simulink model "dsogi_3phpll"  (R2024b)
settings: configuration reference "CONFI" (kept outside this file)
InitFcn:
  | gain_vac=1/(220*sqrt(2));
values from neighbouring files (symbols this model uses):
  cos_th = cos(2*pi*50*t)    [fidelity_pfc_vals.m]
  sin_th = sin(2*pi*50*t)    [fidelity_pfc_vals.m]
  ts = 0.0001    [dic_pfc3ph.sldd]    (also in dictionary.sldd)
  tsw = 1/(fsw*1e3)    (= 1.53846153846e-05)    [fidelity_pfc_vals.m]
undefined symbols (not defined in the file or in its folder): DiscIntNeverNeededParam
libraries: simulink x5, dspswit3 x1, mcbcontrolslib x1
settings Model: DataDictionary=dic_pfc3ph.sldd  Creator=Angel  LastModifiedBy=Angel
settings ConfigSetRef: SourceName=CONFI

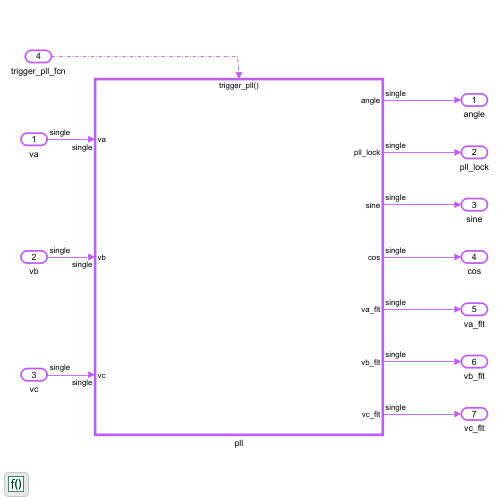
[thumbnail: Simulink's stored preview of the top-level diagram]
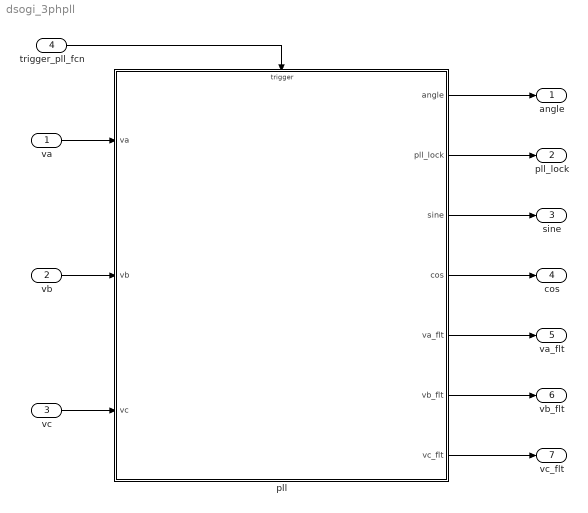
== system dsogi_3phpll ==
  va : Inport  OutDataTypeStr=single
  vb : Inport  Port=2  OutDataTypeStr=single
  vc : Inport  Port=3  OutDataTypeStr=single
  trigger_pll_fcn : Inport  Port=4  OutDataTypeStr=single  OutputFunctionCall=on
  pll : Subsystem
      settings: RTWSystemCode=Inline  RTWFcnNameOpts=Use subsystem name  RTWFileNameOpts=Use subsystem name  RTWMemSecFuncInitTerm=Default  RTWMemSecFuncExecute=Default
  angle : Outport
  pll_lock : Outport  Port=2
  sine : Outport  Port=3
  cos : Outport  Port=4
  va_flt : Outport  Port=5
  vb_flt : Outport  Port=6
  vc_flt : Outport  Port=7
  wires:
  trigger_pll_fcn/1 -> pll/Trigger
  pll/5(va_flt) -> va_flt/1
  va/1 -> pll/1(va)
  pll/2(pll_lock) -> pll_lock/1
  pll/3(sine) -> sine/1
  pll/4(cos) -> cos/1
  vb/1 -> pll/2(vb)
  vc/1 -> pll/3(vc)
  pll/1(angle) -> angle/1
  pll/7(vc_flt) -> vc_flt/1
  pll/6(vb_flt) -> vb_flt/1

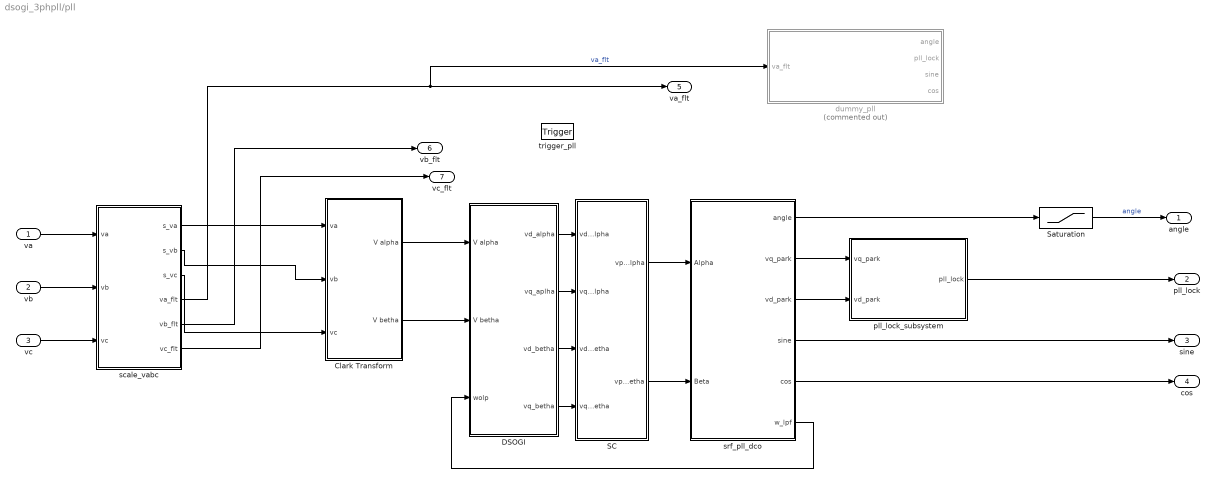
== system dsogi_3phpll/pll ==
  va : Inport  OutDataTypeStr=single
  vb : Inport  Port=2  OutDataTypeStr=single
  vc : Inport  Port=3  OutDataTypeStr=single
  trigger_pll : TriggerPort  TriggerType=function-call  VariantControl=(inherit)  SampleTime=1/10e3  PortDimensions=1
  Clark Transform : Subsystem  SystemSampleTime=ts
  DSOGI : Subsystem  SystemSampleTime=ts
  SC : Subsystem  SystemSampleTime=ts
  Saturation : Saturate  UpperLimit=2*pi  LowerLimit=0
  dummy_pll : Subsystem  Commented=on
  pll_lock_subsystem : Subsystem
  scale_vabc : Subsystem
  srf_pll_dco : Subsystem
  angle : Outport
  pll_lock : Outport  Port=2
  sine : Outport  Port=3
  cos : Outport  Port=4
  va_flt : Outport  Port=5
  vb_flt : Outport  Port=6
  vc_flt : Outport  Port=7
  wires:
  vb/1 -> scale_vabc/2(vb)
  scale_vabc/3(s_vc) -> Clark Transform/3(vc)
  scale_vabc/2(s_vb) -> Clark Transform/2(vb)
  srf_pll_dco/5(cos) -> cos/1
  pll_lock_subsystem/1(pll_lock) -> pll_lock/1
  srf_pll_dco/2(vq_park) -> pll_lock_subsystem/1(vq_park)
  SC/2(vp_betha) -> srf_pll_dco/2(Beta)
  SC/1(vp_alpha) -> srf_pll_dco/1(Alpha)
  DSOGI/2(vq_aplha) -> SC/2(vq_sogi_alpha)
  DSOGI/1(vd_alpha) -> SC/1(vd_sogi_alpha)
  srf_pll_dco/3(vd_park) -> pll_lock_subsystem/2(vd_park)
  srf_pll_dco/6(w_lpf) -> DSOGI/3(wolp)
  va/1 -> scale_vabc/1(va)
  Clark Transform/2(V betha) -> DSOGI/2(V betha)
  scale_vabc/1(s_va) -> Clark Transform/1(va)
  srf_pll_dco/4(sine) -> sine/1
  srf_pll_dco/1(angle) -> Saturation/1
  DSOGI/3(vd_betha) -> SC/3(vd_sogi_betha)
  Clark Transform/1(V alpha) -> DSOGI/1(V alpha)
  DSOGI/4(vq_betha) -> SC/4(vq_sogi_betha)
  vc/1 -> scale_vabc/3(vc)
  scale_vabc/4(va_flt) -> dummy_pll/1(va_flt), va_flt/1  "va_flt"
  scale_vabc/5(vb_flt) -> vb_flt/1
  scale_vabc/6(vc_flt) -> vc_flt/1
  Saturation/1 -> angle/1  "angle"

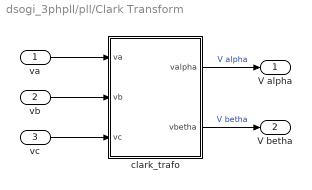
== system dsogi_3phpll/pll/Clark Transform ==
  va : Inport  OutDataTypeStr=single
  vb : Inport  Port=2  OutDataTypeStr=single
  vc : Inport  Port=3  OutDataTypeStr=single
  clark_trafo : MATLAB Function  TreatAsAtomicUnit=on
  V alpha : Outport
  V betha : Outport  Port=2
  wires:
  va/1 -> clark_trafo/1(va)
  vb/1 -> clark_trafo/2(vb)
  vc/1 -> clark_trafo/3(vc)
  clark_trafo/1(valpha) -> V alpha/1  "V alpha"
  clark_trafo/2(vbetha) -> V betha/1  "V betha"

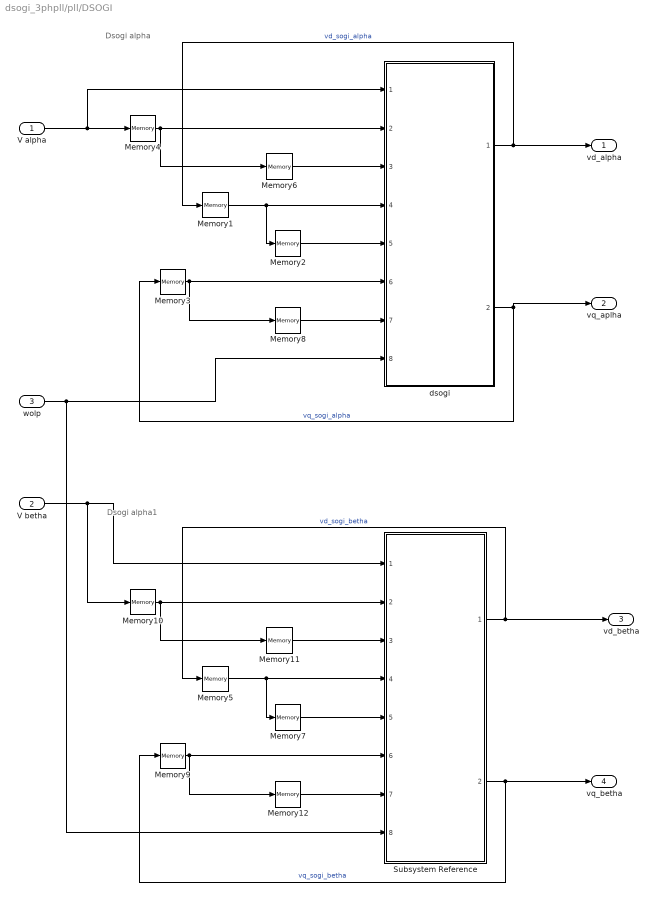
== system dsogi_3phpll/pll/DSOGI ==
  note: Dsogi alpha1
  note: Dsogi alpha
  V alpha : Inport  OutDataTypeStr=single
  V betha : Inport  Port=2  OutDataTypeStr=single
  wolp : Inport  Port=3  OutDataTypeStr=single
  Memory{1..12} (12 alike) : Memory  InheritSampleTime=on
  Subsystem Reference : Subsystem  ReferencedSubsystem=dsogi
  dsogi : Subsystem  ReferencedSubsystem=dsogi
  vd_alpha : Outport
  vq_aplha : Outport  Port=2
  vd_betha : Outport  Port=3
  vq_betha : Outport  Port=4
  wires:
  dsogi/2 -> vq_aplha/1, Memory3/1  "vq_sogi_alpha"
  dsogi/1 -> vd_alpha/1, Memory1/1  "vd_sogi_alpha"
  Memory8/1 -> dsogi/7
  Memory2/1 -> dsogi/5
  Memory6/1 -> dsogi/3
  Memory3/1 -> dsogi/6, Memory8/1
  Memory1/1 -> dsogi/4, Memory2/1
  Memory4/1 -> dsogi/2, Memory6/1
  V alpha/1 -> dsogi/1, Memory4/1
  Subsystem Reference/2 -> vq_betha/1, Memory9/1  "vq_sogi_betha"
  Subsystem Reference/1 -> vd_betha/1, Memory5/1  "vd_sogi_betha"
  wolp/1 -> Subsystem Reference/8, dsogi/8
  Memory12/1 -> Subsystem Reference/7
  Memory7/1 -> Subsystem Reference/5
  Memory11/1 -> Subsystem Reference/3
  V betha/1 -> Subsystem Reference/1, Memory10/1
  Memory10/1 -> Subsystem Reference/2, Memory11/1
  Memory5/1 -> Subsystem Reference/4, Memory7/1
  Memory9/1 -> Subsystem Reference/6, Memory12/1

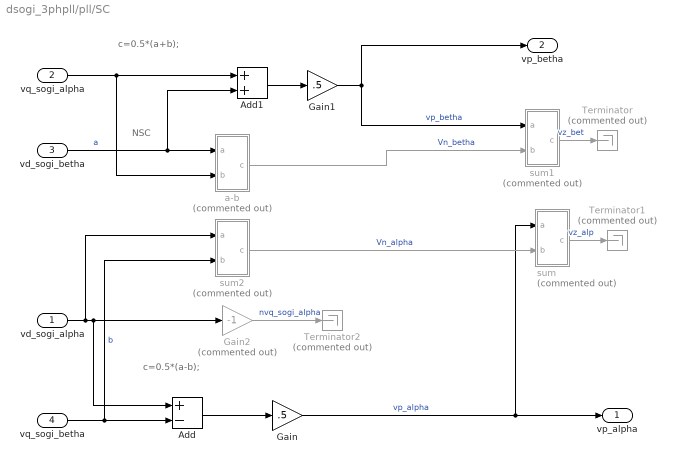
== system dsogi_3phpll/pll/SC ==
  note: c=0.5*(a+b);
  note: c=0.5*(a-b);
  note: NSC
  vd_sogi_alpha : Inport  OutDataTypeStr=single
  vq_sogi_alpha : Inport  Port=2  OutDataTypeStr=single
  vd_sogi_betha : Inport  Port=3  OutDataTypeStr=single
  vq_sogi_betha : Inport  Port=4  OutDataTypeStr=single
  Add : Sum  Inputs=+-
  Add1 : Sum
  Gain : Gain  Gain=.5  OutDataTypeStr=single
  Gain1 : Gain  Gain=.5  OutDataTypeStr=single
  Gain2 : Gain  Commented=on  Gain=-1
  Terminator : Terminator  Commented=on
  Terminator1 : Terminator  Commented=on
  Terminator2 : Terminator  Commented=on
  a-b : MATLAB Function  Commented=on  TreatAsAtomicUnit=on  VariantControl=false()
      settings: RTWSystemCode=Inline
  sum : MATLAB Function  Commented=on  TreatAsAtomicUnit=on  VariantControl=false()
  sum1 : MATLAB Function  Commented=on  TreatAsAtomicUnit=on  VariantControl=false()
  sum2 : MATLAB Function  Commented=on  TreatAsAtomicUnit=on  VariantControl=false()
      settings: RTWSystemCode=Inline
  vp_alpha : Outport
  vp_betha : Outport  Port=2
  wires:
  vd_sogi_betha/1 -> Add1/2, a-b/1(a)  "a"
  Gain1/1 -> vp_betha/1, sum1/1(a)  "vp_betha"
  vd_sogi_alpha/1 -> Add/1, Gain2/1, sum2/1(a)
  sum/1(c) -> Terminator1/1  "vz_alp"
  Add1/1 -> Gain1/1
  vq_sogi_alpha/1 -> Add1/1, a-b/2(b)
  Add/1 -> Gain/1
  Gain/1 -> sum/1(a), vp_alpha/1  "vp_alpha"
  vq_sogi_betha/1 -> Add/2, sum2/2(b)  "b"
  Gain2/1 -> Terminator2/1  "nvq_sogi_alpha"
  sum1/1(c) -> Terminator/1  "vz_bet"
  a-b/1(c) -> sum1/2(b)  "Vn_betha"
  sum2/1(c) -> sum/2(b)  "Vn_alpha"

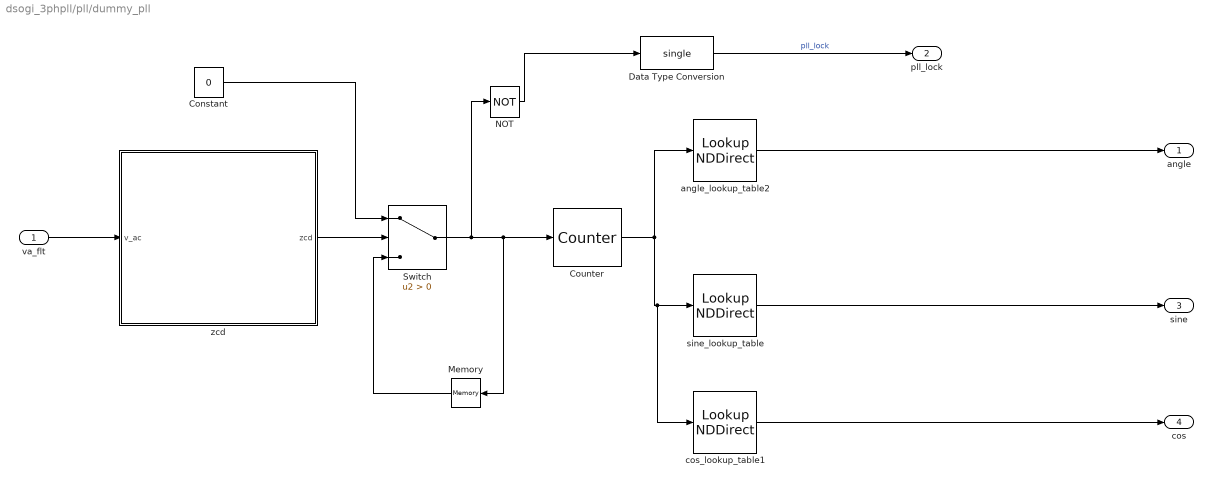
== system dsogi_3phpll/pll/dummy_pll ==
  va_flt : Inport
  Constant : Constant  Value=0  OutDataTypeStr=boolean  SampleTime=-1
  Counter : dspswit3/Counter  Direction=Up  CountEvent=Free running  CounterSize=User defined  MaxCount=200  InitialCount=0  Output=Count  HitValue=32  ResetInput=on  SamplesPerFrame=1  Ts=-1  CntDtype=uint32  HitDtype=Logical
  Data Type Conversion : DataTypeConversion  OutDataTypeStr=single  SaturateOnIntegerOverflow=off  RndMeth=Floor
  Memory : Memory  InitialCondition=1  InheritSampleTime=on
  NOT : Logic  Operator=NOT  IconShape=distinctive  AllPortsSameDT=off  OutDataTypeStr=boolean
  Switch : Switch  Criteria=u2 > Threshold  SaturateOnIntegerOverflow=off  InputSameDT=off
  angle_lookup_table2 : LookupNDDirect  NumberOfTableDimensions=1  Table=single(2*pi*50*t)  RemoveProtectionInput=on
  cos_lookup_table1 : LookupNDDirect  NumberOfTableDimensions=1  Table=single(cos_th)  RemoveProtectionInput=on
  sine_lookup_table : LookupNDDirect  NumberOfTableDimensions=1  Table=single(sin_th)  RemoveProtectionInput=on
  zcd : Subsystem  SystemSampleTime=tsw
  angle : Outport
  pll_lock : Outport  Port=2
  sine : Outport  Port=3
  cos : Outport  Port=4
  wires:
  va_flt/1 -> zcd/1(v_ac)
  Memory/1 -> Switch/3
  Switch/1 -> NOT/1, Counter/1, Memory/1
  zcd/1(zcd) -> Switch/2
  Constant/1 -> Switch/1
  cos_lookup_table1/1 -> cos/1
  sine_lookup_table/1 -> sine/1
  NOT/1 -> Data Type Conversion/1
  Counter/1 -> angle_lookup_table2/1, cos_lookup_table1/1, sine_lookup_table/1
  angle_lookup_table2/1 -> angle/1
  Data Type Conversion/1 -> pll_lock/1  "pll_lock"

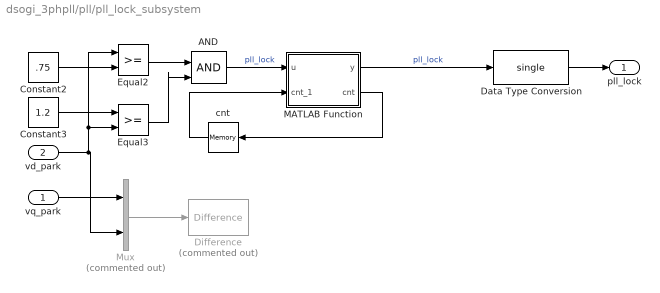
== system dsogi_3phpll/pll/pll_lock_subsystem ==
  vq_park : Inport
  vd_park : Inport  Port=2
  AND : Logic  IconShape=distinctive  AllPortsSameDT=off  OutDataTypeStr=boolean
  Constant2 : Constant  Value=.75  OutDataTypeStr=single  SampleTime=-1
  Constant3 : Constant  Value=1.2  OutDataTypeStr=single  SampleTime=-1
  Data Type Conversion : DataTypeConversion  OutDataTypeStr=single  SaturateOnIntegerOverflow=off  RndMeth=Floor
  Difference : simulink/Discrete/Difference  Commented=on  ICPrevInput=0.0  OutMin=[]  OutMax=[]  OutDataType=fixdt(1, 16)  OutScaling=2^-10  DoSatur=off
  Equal2 : RelationalOperator  OutDataTypeStr=boolean  RndMeth=Simplest  InputSameDT=off
  Equal3 : RelationalOperator  OutDataTypeStr=boolean  RndMeth=Simplest  InputSameDT=off
  MATLAB Function : MATLAB Function  TreatAsAtomicUnit=on
  Mux : Mux  Commented=on  Inputs=2
  cnt : Memory  InheritSampleTime=on
  pll_lock : Outport
  wires:
  Equal3/1 -> AND/2
  Constant2/1 -> Equal2/2
  Constant3/1 -> Equal3/1
  vd_park/1 -> Equal3/2, Equal2/1, Mux/2
  vq_park/1 -> Mux/1
  Equal2/1 -> AND/1
  Mux/1 -> Difference/1
  cnt/1 -> MATLAB Function/2(cnt_1)
  AND/1 -> MATLAB Function/1(u)  "pll_lock"
  MATLAB Function/2(cnt) -> cnt/1
  Data Type Conversion/1 -> pll_lock/1
  MATLAB Function/1(y) -> Data Type Conversion/1  "pll_lock"

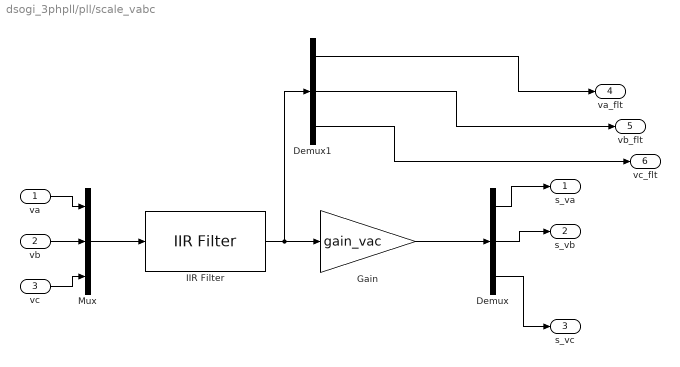
== system dsogi_3phpll/pll/scale_vabc ==
  va : Inport
  vb : Inport  Port=2
  vc : Inport  Port=3
  Demux : Demux  Outputs=3
  Demux1 : Demux  Outputs=3
  Gain : Gain  Gain=gain_vac  OutDataTypeStr=single
  IIR Filter : mcbcontrolslib/IIR Filter  VariantControl=Low Pass Filter  VariantSelect=Low-pass  FilterConstantInputType=Specify via dialog  Filter_constant=.1  advancedSettings=on  Ts=1/8e3  cutOff_freq=141.4711
  Mux : Mux  Inputs=3
  s_va : Outport
  s_vb : Outport  Port=2
  s_vc : Outport  Port=3
  va_flt : Outport  Port=4
  vb_flt : Outport  Port=5
  vc_flt : Outport  Port=6
  wires:
  va/1 -> Mux/1
  Gain/1 -> Demux/1
  vb/1 -> Mux/2
  vc/1 -> Mux/3
  Mux/1 -> IIR Filter/1
  Demux/2 -> s_vb/1
  Demux/1 -> s_va/1
  Demux/3 -> s_vc/1
  IIR Filter/1 -> Demux1/1, Gain/1
  Demux1/1 -> va_flt/1
  Demux1/2 -> vb_flt/1
  Demux1/3 -> vc_flt/1

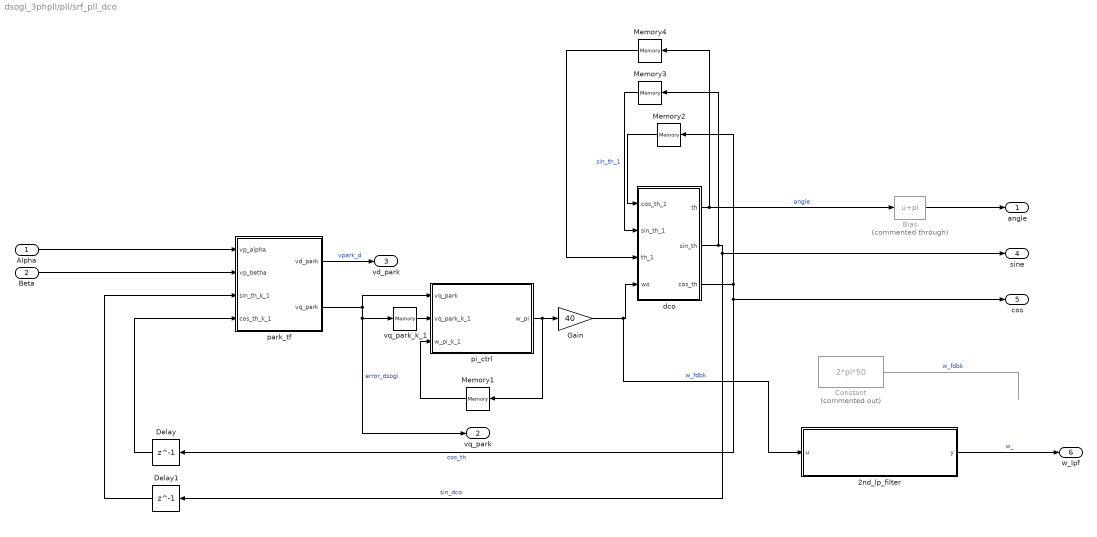
== system dsogi_3phpll/pll/srf_pll_dco ==
  Alpha : Inport  OutDataTypeStr=single
  Beta : Inport  Port=2  OutDataTypeStr=single
  2nd_lp_filter : Subsystem
  Bias : Bias  Commented=through  Bias=pi  SaturateOnIntegerOverflow=off
  Constant : Constant  Commented=on  Value=2*pi*50  OutDataTypeStr=single  SampleTime=-1
  Delay : Delay  DelayLength=1
  Delay1 : Delay  DelayLength=1
  Gain : Gain  Gain=40  OutDataTypeStr=single
  Memory1 : Memory  InheritSampleTime=on
  Memory2 : Memory  InitialCondition=.99  InheritSampleTime=on
  Memory3 : Memory  InheritSampleTime=on
  Memory4 : Memory  InheritSampleTime=on
  dco : MATLAB Function  TreatAsAtomicUnit=on  VariantControl=false()
  park_tf : MATLAB Function  TreatAsAtomicUnit=on  VariantControl=false()
  pi_ctrl : MATLAB Function  TreatAsAtomicUnit=on  VariantControl=false()
  vq_park_k_1 : Memory  InheritSampleTime=on
  angle : Outport
  vq_park : Outport  Port=2
  vd_park : Outport  Port=3
  sine : Outport  Port=4
  cos : Outport  Port=5
  w_lpf : Outport  Port=6
  wires:
  Memory2/1 -> dco/1(cos_th_1)
  Memory1/1 -> pi_ctrl/3(w_pi_k_1)
  dco/1(th) -> Bias/1, Memory4/1  "angle"
  Beta/1 -> park_tf/2(vp_betha)
  Alpha/1 -> park_tf/1(vp_alpha)
  dco/3(cos_th) -> cos/1, Delay/1, Memory2/1  "cos_th"
  park_tf/2(vq_park) -> vq_park/1, vq_park_k_1/1, pi_ctrl/1(vq_park)  "error_dsogi"
  vq_park_k_1/1 -> pi_ctrl/2(vq_park_k_1)
  dco/2(sin_th) -> sine/1, Delay1/1, Memory3/1  "sin_dco"
  park_tf/1(vd_park) -> vd_park/1  "vpark_d"
  Delay1/1 -> park_tf/3(sin_th_k_1)
  Memory4/1 -> dco/3(th_1)
  pi_ctrl/1(w_pi) -> Memory1/1, Gain/1
  Memory3/1 -> dco/2(sin_th_1)  "sin_th_1"
  Delay/1 -> park_tf/4(cos_th_k_1)
  Gain/1 -> 2nd_lp_filter/1(u), dco/4(wo)  "w_fdbk"
  Bias/1 -> angle/1
  Constant/1 -> ?  "w_fdbk"
  2nd_lp_filter/1(y) -> w_lpf/1  "w_"

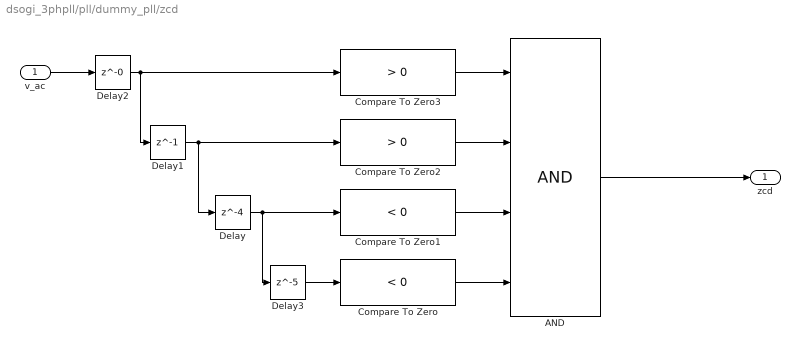
== system dsogi_3phpll/pll/dummy_pll/zcd ==
  v_ac : Inport  OutDataTypeStr=single
  AND : Logic  Inputs=4  AllPortsSameDT=off  OutDataTypeStr=boolean
  Compare To Zero : simulink/Logic and Bit Operations/Compare To Zero  relop=<  OutDataTypeStr=boolean
  Compare To Zero1 : simulink/Logic and Bit Operations/Compare To Zero  relop=<  OutDataTypeStr=boolean
  Compare To Zero2 : simulink/Logic and Bit Operations/Compare To Zero  relop=>  OutDataTypeStr=boolean
  Compare To Zero3 : simulink/Logic and Bit Operations/Compare To Zero  relop=>  OutDataTypeStr=boolean
  Delay : Delay  DelayLength=4
  Delay1 : Delay  DelayLength=1
  Delay2 : Delay  DelayLength=0
  Delay3 : Delay  DelayLength=5
  zcd : Outport
  wires:
  v_ac/1 -> Delay2/1
  Delay3/1 -> Compare To Zero/1
  Delay/1 -> Delay3/1, Compare To Zero1/1
  Delay2/1 -> Compare To Zero3/1, Delay1/1
  Delay1/1 -> Compare To Zero2/1, Delay/1
  Compare To Zero3/1 -> AND/1
  Compare To Zero1/1 -> AND/3
  Compare To Zero/1 -> AND/4
  Compare To Zero2/1 -> AND/2
  AND/1 -> zcd/1

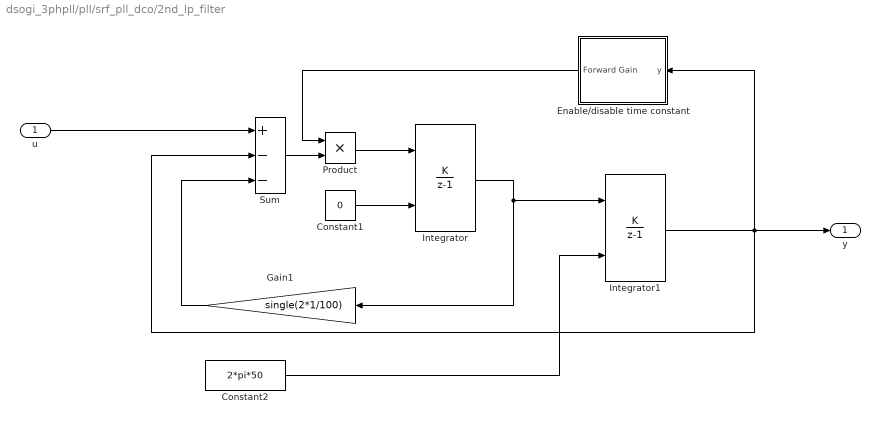
== system dsogi_3phpll/pll/srf_pll_dco/2nd_lp_filter ==
  u : Inport
  Constant1 : Constant  Value=0  OutDataTypeStr=single  SampleTime=-1
  Constant2 : Constant  Value=2*pi*50  OutDataTypeStr=single  SampleTime=-1
  Enable/disable time constant : Subsystem
  Gain1 : Gain  Gain=single(2*1/100)
  Integrator : DiscreteIntegrator  IntegratorMethod=Accumulation: Forward Euler  gainval=1/8e3  InitialConditionSource=external  SampleTime=-1  ICPrevOutput=DiscIntNeverNeededParam  ICPrevScaledInput=DiscIntNeverNeededParam
  Integrator1 : DiscreteIntegrator  IntegratorMethod=Accumulation: Forward Euler  gainval=1/8e3  InitialConditionSource=external  SampleTime=-1  ICPrevOutput=DiscIntNeverNeededParam  ICPrevScaledInput=DiscIntNeverNeededParam
  Product : Product
  Sum : Sum  Inputs=+--
  y : Outport  VectorParamsAs1DForOutWhenUnconnected=off
  wires:
  Integrator1/1 -> y/1, Enable/disable time constant/1(y), Sum/2
  Sum/1 -> Product/2
  Constant2/1 -> Integrator1/2
  Constant1/1 -> Integrator/2
  Integrator/1 -> Integrator1/1, Gain1/1
  u/1 -> Sum/1
  Product/1 -> Integrator/1
  Gain1/1 -> Sum/3
  Enable/disable time constant/1(Forward Gain) -> Product/1

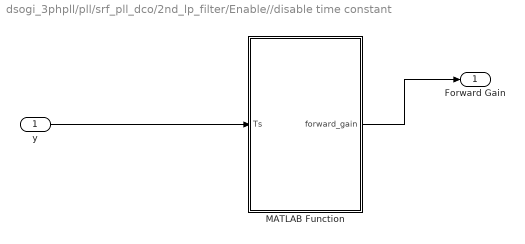
== system dsogi_3phpll/pll/srf_pll_dco/2nd_lp_filter/Enable//disable time constant ==
  y : Inport
  MATLAB Function : MATLAB Function  TreatAsAtomicUnit=on
  Forward Gain : Outport  VectorParamsAs1DForOutWhenUnconnected=off
  wires:
  MATLAB Function/1(forward_gain) -> Forward Gain/1
  y/1 -> MATLAB Function/1(Ts)

== matlab function dsogi_3phpll/pll/pll_lock_subsystem/MATLAB Function ==
  data: u input; y output boolean; cnt_1 input single; cnt output
function [y,cnt] = fcn(u, cnt_1)
y=false;
cnt = cnt_1;
if u == true
   if cnt_1<=single(5*(10e3/50)) 
      cnt = cnt_1 + single(1.0);
      y=false;
   else 
      y=true;
   end
else 
   y=false;
   cnt = single(0.0);
end

== matlab function dsogi_3phpll/pll/srf_pll_dco/2nd_lp_filter/Enable//disable time constant/MATLAB Function ==
  data: Ts input; forward_gain output
function forward_gain  = fcn(Ts)


    forward_gain = single(1/max(Ts,single(1/(100*100))));
   
end

== matlab function dsogi_3phpll/pll/Clark Transform/clark_trafo ==
  data: va input; valpha output; vb input; vc input; vbetha output
function [valpha, vbetha] = clarktrans(va,vb,vc)
tw_thr = single((2/3));
sqrt_3 = single(sqrt(3));
point_5 = single(.5);

valpha=(tw_thr*(va-(point_5*vb)-(point_5*vc)));
vbetha=( (tw_thr*(sqrt_3*point_5))*(vb-vc) );

end

== matlab function dsogi_3phpll/pll/SC/a-b ==
  data: a input; c output; b input
function c = fcn(a,b)

c=0.5*(a-b);
end

== matlab function dsogi_3phpll/pll/SC/sum2 ==
  data: a input; c output; b input
function c = fcn(a,b)

c=0.5*(a+b);
end

== matlab function dsogi_3phpll/pll/SC/sum ==
  data: a input; c output; b input
function c = fcn(a,b)

c=(a-b);
end

== matlab function dsogi_3phpll/pll/SC/sum1 ==
  data: a input; c output; b input
function c = fcn(a,b)

c=(a-b);
end

== matlab function dsogi_3phpll/pll/srf_pll_dco/dco ==
  data: cos_th_1 input single; sin_th_1 input single; th_1 input single; th output single; sin_th output single; wo input single; cos_th output single
function [th,sin_th,cos_th]= dco(cos_th_1,sin_th_1,th_1,wo)
        % ws=(2*pi*50);
        wout=(wo);
        tsample=single(1/8e3);
        %Sin is for showing the overlaping w the input 
        sin_th=sin_th_1+(cos_th_1*wout*tsample); %Sin(t+dt)=sin(t)+cos(t)*dt
        cos_th=cos_th_1-(sin_th_1*wout*tsample);
        
        sin_th=max([sin_th -1]);
        cos_th=max([cos_th -1]);

        sin_th=min([sin_th 1]);
        cos_th=min([cos_th 1]);

        th=th_1+(wout*tsample);

        if sin_th>=0 && sin_th_1<=0
            th=single(0);    %fi(pi,1,32,29); %zero crossing reseting phase angle
        end
      
end

== matlab function dsogi_3phpll/pll/srf_pll_dco/park_tf ==
  data: vd_park output; vp_alpha input; vq_park output; vp_betha input; sin_th_k_1 input; cos_th_k_1 input
  function [vd_park,vq_park] = park(vp_alpha,vp_betha,sin_th_k_1,cos_th_k_1)

vq_park=(sin_th_k_1*vp_betha+cos_th_k_1*vp_alpha);%(-sin_th_k_1*vp_alpha+cos_th_k_1*vp_betha);
vd_park=(sin_th_k_1*vp_alpha-cos_th_k_1*vp_betha);




end

== matlab function dsogi_3phpll/pll/srf_pll_dco/pi_ctrl ==
  data: vq_park input single; w_pi output single; vq_park_k_1 input single; w_pi_k_1 input single
function w_pi = pi_ctrl(vq_park,vq_park_k_1,w_pi_k_1)

fs=single(8e3);
ts=1/fs;
wn_pi=single(100*2*pi);%200*2*pi; 
sig_pi=single(.09);%.05;
vac_peak_pi=single(.3*3.3);

kp =single(2*wn_pi*sig_pi/vac_peak_pi);
ki = single(2*vac_peak_pi/(4*sig_pi*sig_pi));

pi_n1=kp;
pi_n2=(ki*ts)-kp;
sat=single(285);
w_pi=((vq_park)*pi_n1+(vq_park_k_1)*pi_n2+w_pi_k_1);
if (w_pi*40)>single(sat*2*pi)
    w_pi=single(2*85*pi);
end
if (w_pi*40)<single(-sat*2*pi)
    w_pi=single(-2*85*pi);
end

end
